simulink model "SecRwLtStHdrstUpwdDnwdCtrl"  (R2018b)
settings: Solver=FixedStepDiscrete  StartTime=0.0  StopTime=10.0  FixedStep=0.01  RelTol=1e-3
undefined symbols (not defined in the file or in its folder): KeSMSuMdMotFinshdTm_Val, KeSMSuMdRetryTm1_Val, KeSMSuModeReqDurgTm_Val, KeSMSwSecRwLtStHdrstUpwdDnwdEnTrigBitMask_Val
libraries: StCtrlLib x1
settings Model: Creator=sn2xws  LastModifiedBy=sn2xws
settings DataIOCC: SaveFormat=StructureWithTime
settings OptimizationCC: DefaultParameterBehavior=Inlined  EnhancedBackFolding=on  PassReuseOutputArgsAs=Individual arguments  ZeroExternalMemoryAtStartup=off  ZeroInternalMemoryAtStartup=off  OptimizeBlockOrder=speed  DifferentSizesBufferReuse=on  OptimizationCustomize=off
settings DebuggingCC: ParameterTunabilityLossMsg=error
settings ModelReferenceCC: ModelReferenceNumInstancesAllowed=Single
settings SFSimCC: MATLABDynamicMemAlloc=off
settings RTWCC: SystemTargetFile=autosar.tlc  GenCodeOnly=on  TemplateMakefile=ert_default_tmf  Description=AUTOSAR  GenerateReport=on  IncludeHyperlinkInReport=on  LaunchReport=on  GenerateTraceInfo=on  GenerateTraceReport=on  GenerateTraceReportSl=on  GenerateTraceReportSf=on  GenerateTraceReportEml=on
settings CodeAppCC: ForceParamTrailComments=on  IgnoreCustomStorageClasses=off  OperatorAnnotations=on  SimulinkDataObjDesc=on  SFDataObjDesc=on  InsertBlockDesc=on
settings STFCustomTargetCC: TargetLangStandard=C99 (ISO)  MultiwordLength=256  ParMdlRefBuildCompliant=on  CompOptLevelCompliant=on  IncludeMdlTerminateFcn=off  CombineOutputUpdateFcns=on  SuppressErrorStatus=on  ERTCustomFileBanners=on  SupportNonFinite=off  SupportComplex=off  SupportContinuousTime=off  SupportNonInlinedSFcns=off  RemoveResetFunc=on  MATLABClassNameForMDSCustomization=Simulink.SoftwareTarget.ERTCustomization  AutosarCompliant=on  UseToolchainInfoCompliant=on  LookupTableObjectStructAxisOrder=2,1,3,4,...  LUTObjectStructOrderEvenSpacing=Size,Table,Breakpoints  SystemTargetFile=autosar.tlc
settings ERTTargetCC: TargetLangStandard=C99 (ISO)  ConcurrentExecutionCompliant=off  IncludeMdlTerminateFcn=off  SuppressErrorStatus=on  SupportNonFinite=off  SupportComplex=off  ModelStepFunctionPrototypeControlCompliant=off  CPPClassGenCompliant=off  AutosarCompliant=on  LookupTableObjectStructAxisOrder=2,1,3,4,...  LUTObjectStructOrderEvenSpacing=Size,Table,Breakpoints  InlinedParameterPlacement=NonHierarchical  ERTCustomFileTemplate=example_file_process.tlc  ERTFilePackagingFormat=Compact

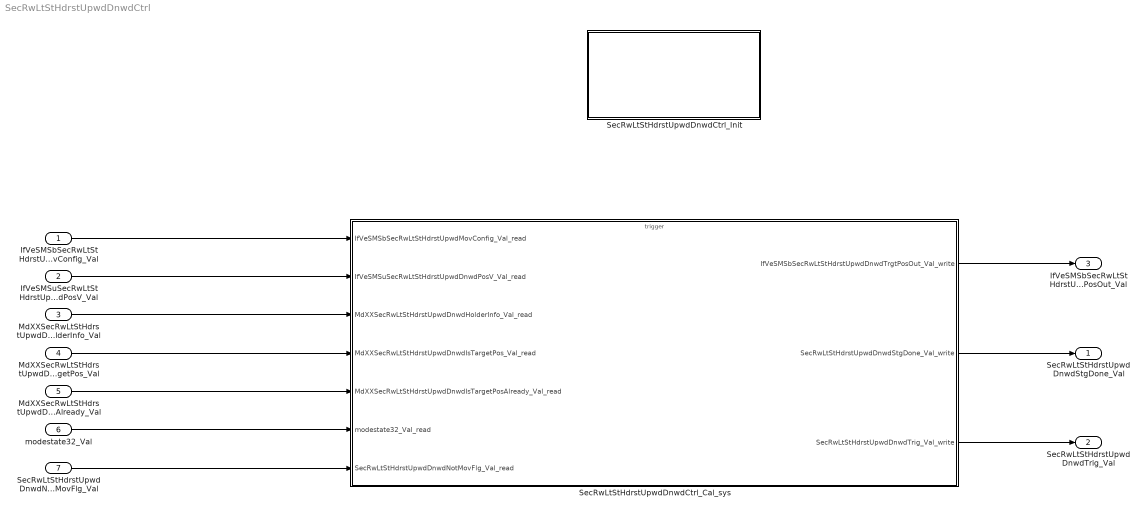
== system SecRwLtStHdrstUpwdDnwdCtrl ==
  IfVeSMSbSecRwLtStHdrstUpwdMovConfig_Val : Inport  OutDataTypeStr=boolean  PortDimensions=1
  IfVeSMSuSecRwLtStHdrstUpwdDnwdPosV_Val : Inport  Port=2  OutDataTypeStr=boolean  PortDimensions=1
  MdXXSecRwLtStHdrstUpwdDnwdHolderInfo_Val : Inport  Port=3  OutDataTypeStr=uint32  PortDimensions=1
  MdXXSecRwLtStHdrstUpwdDnwdIsTargetPos_Val : Inport  Port=4  OutDataTypeStr=uint32  PortDimensions=1
  MdXXSecRwLtStHdrstUpwdDnwdIsTargetPosAlready_Val : Inport  Port=5  OutDataTypeStr=uint32  PortDimensions=1
  modestate32_Val : Inport  Port=6  OutDataTypeStr=uint32  PortDimensions=1
  SecRwLtStHdrstUpwdDnwdNotMovFlg_Val : Inport  Port=7  OutDataTypeStr=boolean  PortDimensions=1
  SecRwLtStHdrstUpwdDnwdCtrl_Cal_sys : Subsystem
  SecRwLtStHdrstUpwdDnwdCtrl_Init : Subsystem
  SecRwLtStHdrstUpwdDnwdStgDone_Val : Outport  OutDataTypeStr=boolean  PortDimensions=1
  SecRwLtStHdrstUpwdDnwdTrig_Val : Outport  Port=2  OutDataTypeStr=boolean  PortDimensions=1
  IfVeSMSbSecRwLtStHdrstUpwdDnwdTrgtPosOut_Val : Outport  Port=3  OutDataTypeStr=boolean  PortDimensions=1
  wires:
  IfVeSMSbSecRwLtStHdrstUpwdMovConfig_Val/1 -> SecRwLtStHdrstUpwdDnwdCtrl_Cal_sys/1(IfVeSMSbSecRwLtStHdrstUpwdMovConfig_Val_read)
  IfVeSMSuSecRwLtStHdrstUpwdDnwdPosV_Val/1 -> SecRwLtStHdrstUpwdDnwdCtrl_Cal_sys/2(IfVeSMSuSecRwLtStHdrstUpwdDnwdPosV_Val_read)
  MdXXSecRwLtStHdrstUpwdDnwdHolderInfo_Val/1 -> SecRwLtStHdrstUpwdDnwdCtrl_Cal_sys/3(MdXXSecRwLtStHdrstUpwdDnwdHolderInfo_Val_read)
  MdXXSecRwLtStHdrstUpwdDnwdIsTargetPos_Val/1 -> SecRwLtStHdrstUpwdDnwdCtrl_Cal_sys/4(MdXXSecRwLtStHdrstUpwdDnwdIsTargetPos_Val_read)
  MdXXSecRwLtStHdrstUpwdDnwdIsTargetPosAlready_Val/1 -> SecRwLtStHdrstUpwdDnwdCtrl_Cal_sys/5(MdXXSecRwLtStHdrstUpwdDnwdIsTargetPosAlready_Val_read)
  modestate32_Val/1 -> SecRwLtStHdrstUpwdDnwdCtrl_Cal_sys/6(modestate32_Val_read)
  SecRwLtStHdrstUpwdDnwdNotMovFlg_Val/1 -> SecRwLtStHdrstUpwdDnwdCtrl_Cal_sys/7(SecRwLtStHdrstUpwdDnwdNotMovFlg_Val_read)
  SecRwLtStHdrstUpwdDnwdCtrl_Cal_sys/1(IfVeSMSbSecRwLtStHdrstUpwdDnwdTrgtPosOut_Val_write) -> IfVeSMSbSecRwLtStHdrstUpwdDnwdTrgtPosOut_Val/1
  SecRwLtStHdrstUpwdDnwdCtrl_Cal_sys/2(SecRwLtStHdrstUpwdDnwdStgDone_Val_write) -> SecRwLtStHdrstUpwdDnwdStgDone_Val/1
  SecRwLtStHdrstUpwdDnwdCtrl_Cal_sys/3(SecRwLtStHdrstUpwdDnwdTrig_Val_write) -> SecRwLtStHdrstUpwdDnwdTrig_Val/1

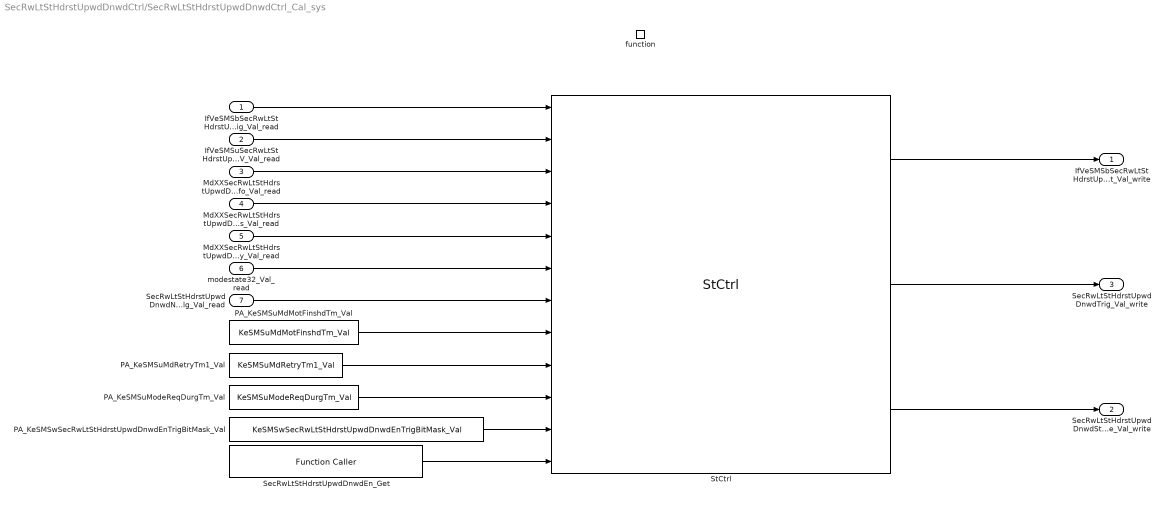
== system SecRwLtStHdrstUpwdDnwdCtrl/SecRwLtStHdrstUpwdDnwdCtrl_Cal_sys ==
  IfVeSMSbSecRwLtStHdrstUpwdMovConfig_Val_read : Inport
  IfVeSMSuSecRwLtStHdrstUpwdDnwdPosV_Val_read : Inport  Port=2
  MdXXSecRwLtStHdrstUpwdDnwdHolderInfo_Val_read : Inport  Port=3
  MdXXSecRwLtStHdrstUpwdDnwdIsTargetPos_Val_read : Inport  Port=4
  MdXXSecRwLtStHdrstUpwdDnwdIsTargetPosAlready_Val_read : Inport  Port=5
  modestate32_Val_read : Inport  Port=6
  SecRwLtStHdrstUpwdDnwdNotMovFlg_Val_read : Inport  Port=7
  function : TriggerPort  TriggerType=function-call  IsSimulinkFunction=on  FunctionName=SecRwLtStHdrstUpwdDnwdCtrl_Cal  VariantControl=(inherit)
  PA_KeSMSuMdMotFinshdTm_Val : Constant  Value=KeSMSuMdMotFinshdTm_Val
  PA_KeSMSuMdRetryTm1_Val : Constant  Value=KeSMSuMdRetryTm1_Val
  PA_KeSMSuModeReqDurgTm_Val : Constant  Value=KeSMSuModeReqDurgTm_Val
  PA_KeSMSwSecRwLtStHdrstUpwdDnwdEnTrigBitMask_Val : Constant  Value=KeSMSwSecRwLtStHdrstUpwdDnwdEnTrigBitMask_Val
  SecRwLtStHdrstUpwdDnwdEn_Get : FunctionCaller  FunctionPrototype=data = SecRwLtStHdrstUpwdDnwdEn_Get()  OutputArgumentSpecifications=uint32(1)
  StCtrl : StCtrlLib/StCtrl  SystemSampleTime=-1
  IfVeSMSbSecRwLtStHdrstUpwdDnwdTrgtPosOut_Val_write : Outport
      settings: EnsureOutportIsVirtual=on
  SecRwLtStHdrstUpwdDnwdStgDone_Val_write : Outport  Port=2
      settings: EnsureOutportIsVirtual=on
  SecRwLtStHdrstUpwdDnwdTrig_Val_write : Outport  Port=3
      settings: EnsureOutportIsVirtual=on
  wires:
  PA_KeSMSwSecRwLtStHdrstUpwdDnwdEnTrigBitMask_Val/1 -> StCtrl/11
  SecRwLtStHdrstUpwdDnwdEn_Get/1 -> StCtrl/12
  PA_KeSMSuMdMotFinshdTm_Val/1 -> StCtrl/8
  PA_KeSMSuModeReqDurgTm_Val/1 -> StCtrl/10
  PA_KeSMSuMdRetryTm1_Val/1 -> StCtrl/9
  IfVeSMSbSecRwLtStHdrstUpwdMovConfig_Val_read/1 -> StCtrl/1
  IfVeSMSuSecRwLtStHdrstUpwdDnwdPosV_Val_read/1 -> StCtrl/2
  MdXXSecRwLtStHdrstUpwdDnwdHolderInfo_Val_read/1 -> StCtrl/3
  MdXXSecRwLtStHdrstUpwdDnwdIsTargetPos_Val_read/1 -> StCtrl/4
  MdXXSecRwLtStHdrstUpwdDnwdIsTargetPosAlready_Val_read/1 -> StCtrl/5
  modestate32_Val_read/1 -> StCtrl/6
  SecRwLtStHdrstUpwdDnwdNotMovFlg_Val_read/1 -> StCtrl/7
  StCtrl/1 -> IfVeSMSbSecRwLtStHdrstUpwdDnwdTrgtPosOut_Val_write/1
  StCtrl/3 -> SecRwLtStHdrstUpwdDnwdStgDone_Val_write/1
  StCtrl/2 -> SecRwLtStHdrstUpwdDnwdTrig_Val_write/1

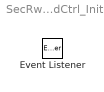
== system SecRwLtStHdrstUpwdDnwdCtrl/SecRwLtStHdrstUpwdDnwdCtrl_Init ==
  Event Listener : EventListener  EventName=reset
